simulink library "FlightGearLib"  (R2021b)
settings: Solver=VariableStepAuto  StartTime=0.0  StopTime=10.0  RelTol=1e-3
undefined symbols (not defined in the file or in its folder): uavData
libraries: aerolibfltsims x2
settings Model: Creator=promero  LastModifiedBy=promero
settings SolverCC: AlgebraicLoopSolver=TrustRegion
settings DebuggingCC: SFMachineParentedDataDiag=warning
settings SFSimCC: CustomCodeUndefinedFunction=UseInterfaceOnly

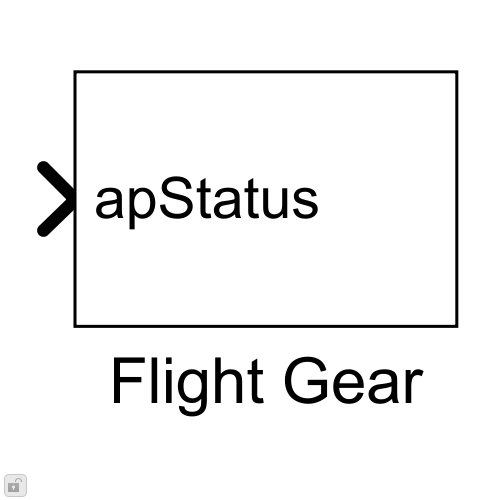
[thumbnail: Simulink's stored preview of the top-level diagram]
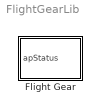
== system FlightGearLib ==
  Flight Gear : Subsystem  VariantControl=animMode == 2

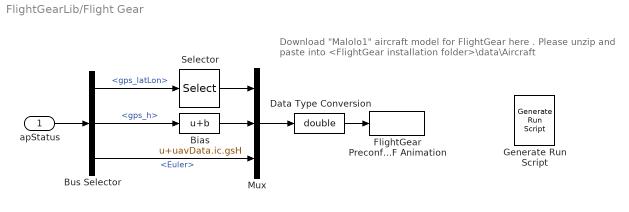
== system FlightGearLib/Flight Gear ==
  note: Download "Malolo1" aircraft model for FlightGear here .
      |
      | Please unzip and paste into <FlightGear installation folder>\data\Aircraft
  apStatus : Inport
  Bias : Bias  Bias=uavData.ic.gsH
  Bus Selector : BusSelector  OutputSignals=gps_latLon,gps_h,Euler
  Data Type Conversion : DataTypeConversion  OutDataTypeStr=double
  FlightGear Preconfigured 6DoF Animation : aerolibfltsims/FlightGear Preconfigured 6DoF Animation  xFlightGearVersion=v2019.1  DestinationIpAddress=127.0.0.1  DestinationPort=5502  SampleTime=1/30  packetVersion=24
  Generate Run Script : aerolibfltsims/Generate Run Script  Architecture=Default  dataFlow=Send  GeometryModelName=Malolo1  AirportId=BOS  RunwayId=10L  InitialAltitude=uavData.ic.Pos_0(3)/0.3048  InitialHeading=uavData.ic.Euler_0(3)*180/pi  OffsetDistance=4.72  OffsetAzimuth=0  InstallScenery=on  DisableShaders=off  OriginAddress=127.0.0.1  DestinationPort=5502  OriginPort=5505  LocalAddress=127.0.0.1  OutputFileName=runfg.bat  FlightGearBaseDirectory=C:\Program Files\FlightGear 2019.1.2
  Mux : Mux  Inputs=3
  Selector : Selector  InputPortWidth=2  IndexOptions=Index vector (dialog)  Indices=[2 1]  OutputSizes=1
  wires:
  Mux/1 -> Data Type Conversion/1
  apStatus/1 -> Bus Selector/1
  Bus Selector/3 -> Mux/3  "<Euler>"
  Data Type Conversion/1 -> FlightGear Preconfigured 6DoF Animation/1
  Bus Selector/1 -> Selector/1  "<gps_latLon>"
  Selector/1 -> Mux/1
  Bus Selector/2 -> Bias/1  "<gps_h>"
  Bias/1 -> Mux/2
